simulink model "proc_control"  (R2024b)
settings: Solver=FixedStepAuto  StartTime=0.0  StopTime=inf  RelTol=1e-3
InitFcn:
  | InitProcControl;
model workspace (MAT data in the model file):
  SL_ROS_VariableLengthArrays_MaxSizes : object (value not decoded)
values from neighbouring files (symbols this model uses):
  A = T200Spec16V{:,3}    [InitProcControl.m]
  dmax = simulation.drift.nominal .* rand(1,6)    [InitProcControl.m]
  dmin = -simulation.drift.nominal .* rand(1,6)    [InitProcControl.m]
  dSeedX = round(rand*10)    [InitProcControl.m]
  dts = 5    [InitProcControl.m]
  N = T200Spec16V{:,6}    [InitProcControl.m]
  PWM = T200Spec16V{:,1}    [InitProcControl.m]
  RPM = T200Spec16V{:,2}    [InitProcControl.m]
undefined symbols (not defined in the file or in its folder): angular_velocity, current_gains, data, data_SL_Info, DiscIntNeverNeededParam, elevation, heading, is_mpc_alive, is_trajectory_done, linear_acceleration, motor1, motor2, motor3, motor4, motor5, motor6, motor7, motor8, MPC, mpc_mode, mpc_status, orientation, physics, pose, position, simulation, simulink, target_reached, thrusters_status, thrusters_status_SL_Info, twist, x_vel_btm, y_vel_btm, z_vel_btm
libraries: ros2lib x85, aerolibutil x12, simulink x9, mpclib x3, embmathops x2, sharedtransform x2, robotcorelib x2, sharedTrackingLibrary x1
(part 2 of 3)

== system proc_control/Subsystem Controller/If Action Subsystem ==
  mode : Inport
  mo : Inport  Port=2
  Current : Inport  Port=3
  mpcParams : Inport  Port=4
  Action Port : ActionPort  InitializeStates=reset  ActionPortLabel=if(u1 >= 0)
  Bus Creator : BusCreator  Inputs=9
  Bus Selector : BusSelector  OutputSignals=qS2W
  Bus Selector1 : BusSelector  OutputSignals=data
  Constant : Constant  Commented=on  Value=false
  MATLAB System : MATLABSystem  System=mpcManager  mpcConst=MPC  mode=mode  SimulateUsing=Code generation
      mask Type: mpcManager
      mask Display:
      | disp('mpcManager');
      | port_label('input',1,'newRosGains');
      | port_label('input',2,'rosGains');
      | port_label('input',3,'mode');
      | port_label('input',4,'newReadCurrent');
      | port_label('input',5,'readCurrent');
      | port_label('input',6,'estimatedCurrent');
      | port_label('input',7,'mo');
      | port_label('input',8,'mpcParams');
      | port_label('output',1,'mvmin');
      | port_label('output',2,'mvmax');
      | port_label('output',3,'ywt');
      | port_label('output',4,'mvwt');
      | port_label('output',5,'dmwwt');
      | port_label('output',6,'tInfo');
      | port_label('output',7,'kill');
      | port_label('output',8,'p');
      | port_label('output',9,'m');
  Subscribe : ros2lib/Subscribe  topicSource=Specify your own  topic=/proc_control/set_mpc_gains  messageType=sonia_common_ros2/MpcGains  sampleTime=inf  QOSHistory=Keep last  QOSDepth=1  QOSReliability=Reliable  QOSDurability=Volatile  QOSDeadline=5  QOSLifespan=5  QOSLiveliness=Automatic  QOSLeaseDuration=5  QOSAvoidROSNamespaceConventions=off
  Subscribe1 : ros2lib/Subscribe  topicSource=Specify your own  topic=/provider_power/current_not  messageType=std_msgs/Float64MultiArray  sampleTime=-1  QOSHistory=Keep last  QOSDepth=1  QOSReliability=Reliable  QOSDurability=Volatile  QOSDeadline=5  QOSLifespan=5  QOSLiveliness=Automatic  QOSLeaseDuration=5  QOSAvoidROSNamespaceConventions=off
  Subsystem : Subsystem  Commented=on
  Transpose : Math  Operator=transpose
  MPC param : Outport
  wires:
  mode/1 -> MATLAB System/3
  Current/1 -> MATLAB System/6
  mo/1 -> Bus Selector/1
  Transpose/1 -> MATLAB System/5
  Bus Selector1/1 -> Transpose/1  "<data>"
  Bus Selector/1 -> MATLAB System/7  "<qS2W>"
  MATLAB System/1 -> Bus Creator/1  "mvmin"
  MATLAB System/2 -> Bus Creator/2  "mvmax"
  MATLAB System/3 -> Bus Creator/3  "ywt"
  MATLAB System/4 -> Bus Creator/4  "mvwt"
  MATLAB System/5 -> Bus Creator/5  "dmwwt"
  MATLAB System/6 -> Bus Creator/6  "thrustersStatus"
  MATLAB System/7 -> Bus Creator/7  "kill"
  MATLAB System/8 -> Bus Creator/8  "p"
  MATLAB System/9 -> Bus Creator/9  "m"
  Bus Creator/1 -> MPC param/1
  mpcParams/1 -> MATLAB System/8
  Subscribe1/2 -> Bus Selector1/1  "data"
  Subscribe1/1 -> MATLAB System/4
  Subscribe/2 -> MATLAB System/2
  Subscribe/1 -> MATLAB System/1

== system proc_control/Subsystem Controller/Post Traitement ==
  In1 : Inport
  MpcParams : Inport  Port=2
  Bus Creator : BusCreator  Inputs=6
  Bus Selector : BusSelector  OutputSignals=mv
  Bus Selector1 : BusSelector  OutputSignals=mvmax,mvmin
  Bus Selector2 : BusSelector  OutputSignals=MpcStatus
  Bus Selector3 : BusSelector  OutputSignals=alive
  Data Type Conversion : DataTypeConversion  OutDataTypeStr=boolean  SaturateOnIntegerOverflow=off  RndMeth=Floor
  Delay : Delay  DelayLength=1  SampleTime=MPC.Ts
  N to A : Lookup_n-D  NumberOfTableDimensions=1  BreakpointsForDimension1=N  BreakpointsForDimension3=[5, 7]  BeginIndexSearchUsingPreviousIndexResult=on  Table=A  InterpMethod=Nearest  DiagnosticForOutOfRangeInput=Warning  RemoveProtectionInput=on  InternalRulePriority=Speed  OutDataTypeStr=uint16  RndMeth=Simplest
  PSU Safe : simulink/Discontinuities/Saturation Dynamic  OutMin=[]  OutMax=[]  OutDataTypeStr=Inherit: Same as second input  OutDataType=fixdt(1, 16)  OutScaling=2^-10  DoSatur=off
  Sum : Sum  Inputs=|+-
  Transpose : Math  Operator=transpose
  n-D Lookup Table1 : Lookup_n-D  NumberOfTableDimensions=1  BreakpointsForDimension1=N  BreakpointsForDimension3=[5, 7]  BeginIndexSearchUsingPreviousIndexResult=on  Table=PWM  InterpMethod=Nearest  DiagnosticForOutOfRangeInput=Warning  RemoveProtectionInput=on  InternalRulePriority=Speed  OutDataTypeStr=uint16  RndMeth=Simplest
  out : Outport
  wires:
  In1/1 -> Bus Selector3/1, Bus Selector2/1, Bus Selector/1
  Bus Selector/1 -> Transpose/1  "<mv>"
  Transpose/1 -> PSU Safe/2
  Bus Selector1/1 -> PSU Safe/1  "<mvmax>"
  Bus Selector1/2 -> PSU Safe/3  "<mvmin>"
  PSU Safe/1 -> N to A/1, n-D Lookup Table1/1, Bus Creator/3  "Newton"
  n-D Lookup Table1/1 -> Bus Creator/2  "pwm"
  N to A/1 -> Bus Creator/1  "current"
  MpcParams/1 -> Bus Creator/4, Bus Selector1/1  "mpcParams"
  Bus Selector2/1 -> Bus Creator/5  "<MpcStatus>"
  Bus Selector3/1 -> Sum/2, Delay/1  "<alive>"
  Delay/1 -> Sum/1
  Sum/1 -> Data Type Conversion/1
  Data Type Conversion/1 -> Bus Creator/6  "isMpcAlive"
  Bus Creator/1 -> out/1

== system proc_control/Subsystem ProcNav/AHRS//Detph Mesurments ==
  note: Modified with Zac
  note: REVIEW
  note: mettre le quaternion dans
      | le W frame
  y : Inport
  Bus Selector : BusSelector  OutputSignals=VN IMU Quaternion  OutputAsBus=on
  Bus Selector1 : BusSelector  OutputSignals=VN IMU Linear Acc  OutputAsBus=on
  Bus Selector2 : BusSelector  OutputSignals=VN IMU Angular Rate  OutputAsBus=on
  Constant : Constant  Value=simulation.sensors.imu.acc.bias
  Discrete-Time Integrator : DiscreteIntegrator  IntegratorMethod=Integration: Trapezoidal  SampleTime=-1  ICPrevOutput=DiscIntNeverNeededParam  ICPrevScaledInput=DiscIntNeverNeededParam
  MATLAB Function : MATLAB Function  TreatAsAtomicUnit=on
  Mux : Mux  Inputs=2
  Quaternion Conjugate : aerolibutil/Quaternion Conjugate
  Quaternion Inverse : aerolibutil/Quaternion Inverse
  Quaternion Rotation : aerolibutil/Quaternion Rotation
  Quaternion Rotation1 : aerolibutil/Quaternion Rotation
  Sum : Sum  Inputs=-+|
  IMU : Outport
  wires:
  y/1 -> Bus Selector2/1, Bus Selector1/1, Bus Selector/1
  Bus Selector/1 -> MATLAB Function/1(u), Quaternion Rotation1/1
  MATLAB Function/1(y) -> Quaternion Conjugate/1
  Quaternion Conjugate/1 -> Quaternion Rotation/1, Quaternion Inverse/1
  Quaternion Inverse/1 -> Mux/1  "qS2W"
  Quaternion Rotation1/1 -> Sum/1
  Bus Selector1/1 -> Quaternion Rotation/2, Sum/2
  Constant/1 -> Quaternion Rotation1/2
  Bus Selector2/1 -> Mux/2  "Angular Rate"
  Sum/1 -> Discrete-Time Integrator/1
  Mux/1 -> IMU/1

== system proc_control/Subsystem ProcNav/DVL Measurements ==
  note: Mettre les vitesse dvl dans le frame Sous-marin
  DVL Velocity : Inport
  mecConst : Inport  Port=2
  Enable : EnablePort
  Bus Creator : BusCreator  Inputs=3
  Bus Selector : BusSelector  OutputSignals=dvl_rotation
  Bus Selector1 : BusSelector  OutputSignals=DVL Bot Velocity
  Bus Selector2 : BusSelector  OutputSignals=DVL Water Velocity
  Constant : Constant  Value=simulation.sensors.dvl.maxSpeedThres
  DVL2Ship : Subsystem
  MATLAB Function : MATLAB Function  TreatAsAtomicUnit=on
  Quaternion Rotation : aerolibutil/Quaternion Rotation
  Scope : Scope
  DVL Measurements : Outport
  wires:
  mecConst/1 -> Bus Selector/1
  DVL Velocity/1 -> Bus Selector1/1, Bus Selector2/1
  Bus Selector/1 -> DVL2Ship/1(dvl Rotation)  "<dvl_rotation>"
  Bus Selector1/1 -> MATLAB Function/1(vBot)  "<DVL Bot Velocity>"
  Bus Selector2/1 -> MATLAB Function/2(vWater)  "<DVL Water Velocity>"
  Constant/1 -> MATLAB Function/3(thres)
  MATLAB Function/1(v) -> Quaternion Rotation/2
  DVL2Ship/1(Quat) -> Quaternion Rotation/1
  Quaternion Rotation/1 -> Bus Creator/1, Scope/1  "Body Velocity"
  MATLAB Function/2(error) -> Bus Creator/2  "error"
  MATLAB Function/3(enable) -> Bus Creator/3  "enable"
  Bus Creator/1 -> DVL Measurements/1

== system proc_control/Subsystem ProcNav/Depth Measurements ==
  note: Transformer la mesure du detph selon BF
  y : Inport
  mecConst : Inport  Port=2
  xhat : Inport  Port=3
  Enable : EnablePort
  Bus Selector : BusSelector  OutputSignals=Pressure Depth  OutputAsBus=on
  Bus Selector1 : BusSelector  OutputSignals=depth_pose
  Discrete Transfer Fcn : DiscreteTransferFcn  Numerator=[physics.thruster.a1 0 ]  Denominator="[1  physics.thruster.b0]"
  Discrete Derivative : simulink/Discrete/Discrete Derivative  gainval=1.0  ICPrevScaledInput=0.0  OutMin=[]  OutMax=[]  OutDataType=fixdt(1, 16)  OutScaling=2^-10  DoSatur=off
  Mux : Mux  Inputs=2
  Quaternion Rotation : aerolibutil/Quaternion Rotation
  Selector : Selector  InputPortWidth=7  IndexOptions=Index vector (dialog)  Indices=[1:4]  OutputSizes=1
  Selector1 : Selector  InputPortWidth=3  IndexOptions=Index vector (dialog)  Indices=[3]  OutputSizes=1
  Sum : Sum  Inputs=|+-
  Depth Measurements : Outport
  wires:
  y/1 -> Bus Selector/1
  Bus Selector/1 -> Sum/1  "pressure Depth"
  Sum/1 -> Mux/1, Discrete Derivative/1  "z position"
  xhat/1 -> Selector/1
  mecConst/1 -> Bus Selector1/1
  Selector/1 -> Quaternion Rotation/1
  Bus Selector1/1 -> Quaternion Rotation/2  "<depth_pose>"
  Quaternion Rotation/1 -> Selector1/1
  Selector1/1 -> Sum/2
  Mux/1 -> Depth Measurements/1
  Discrete Derivative/1 -> Discrete Transfer Fcn/1
  Discrete Transfer Fcn/1 -> Mux/2  "z velocity"

== system proc_control/Subsystem ProcNav/Enabled Subsystem ==
  stateFuncArguments : Inport
  AHRS Mesurments : Inport  Port=2
  "DVL Measurements " : Inport  Port=3
  Depth Measurements : Inport  Port=4
  mecConst : Inport  Port=5
  SLAM VIS : Inport  Port=6
  Enable : EnablePort  StatesWhenEnabling=reset
  Bus Selector : BusSelector  OutputSignals=dvl_lost_override
  Bus Selector1 : BusSelector  OutputSignals=enable,Body Velocity
  Bus Selector2 : BusSelector  OutputSignals=VisIsEnabled,VisData
  Constant : Constant
  Constant1 : Constant  Value=false
  Extended Kalman Filter : sharedTrackingLibrary/Extended Kalman Filter  StateTransitionFcn=EkfNavStatesEq  HasStateTransitionJacobianFcn=off  HasAdditiveProcessNoise=Additive  ProcessNoise=kalman.Cx  HasTimeVaryingProcessNoise=off  HasStateTransitionFcnExtraArgument=1  InitialState=kalman.Xi  InitialStateCovariance=kalman.Ci  MeasurementFcn1=EkfNavAhrs  HasMeasurementJacobianFcn1=off  HasMeasurementEnablePort1=off  HasAdditiveMeasurementNoise1=Additive  MeasurementNoise1=kalman.Cimu  HasTimeVaryingMeasurementNoise1=off  HasMeasurementFcnExtraArgument1=0  HasMeasurementWrapping1=off  MeasurementFcn2=EkfNavDvl  HasMeasurementJacobianFcn2=off  HasMeasurementEnablePort2=on  HasAdditiveMeasurementNoise2=Additive  MeasurementNoise2=kalman.Cdvl  HasTimeVaryingMeasurementNoise2=off  HasMeasurementFcnExtraArgument2=0  HasMeasurementWrapping2=off  MeasurementFcn3=EkfNavDepth  HasMeasurementJacobianFcn3=off  HasMeasurementEnablePort3=off  HasAdditiveMeasurementNoise3=Additive  MeasurementNoise3=kalman.Cdepth  HasTimeVaryingMeasurementNoise3=off  HasMeasurementFcnExtraArgument3=0  HasMeasurementWrapping3=off  MeasurementFcn4=EkfNavSlamVis  HasMeasurementJacobianFcn4=off  HasMeasurementEnablePort4=on  HasAdditiveMeasurementNoise4=Additive  MeasurementNoise4=kalman.CslamVis  HasTimeVaryingMeasurementNoise4=off  HasMeasurementFcnExtraArgument4=0  HasMeasurementWrapping4=off  MeasurementFcn5=EkfNavSlamTracking  HasMeasurementJacobianFcn5=off  HasMeasurementEnablePort5=on  HasAdditiveMeasurementNoise5=Additive  MeasurementNoise5=kalman.CslamTracking  HasTimeVaryingMeasurementNoise5=off  HasMeasurementFcnExtraArgument5=0  HasMeasurementWrapping5=off  EnableMultirate=on  StateTransitionFcnSampleTime=simulink.procNav.sampletime  MeasurementFcn1SampleTime=simulink.procNav.imuDepth.sampletime  MeasurementFcn2SampleTime=simulink.procNav.dvl.sampletime  MeasurementFcn3SampleTime=simulation.sensors.depth.sampletime  MeasurementFcn4SampleTime=0.1  MeasurementFcn5SampleTime=0.1  UseCurrentEstimator=on  OutputStateCovariance=off  DataType=double  SampleTime=1  NumberOfMeasurements=4
  Switch : Switch  Criteria=u2 > Threshold  SaturateOnIntegerOverflow=off  InputSameDT=off
  Zero-Order Hold : ZeroOrderHold  SampleTime=simulink.procNav.dvl.sampletime
  Zero-Order Hold1 : ZeroOrderHold  SampleTime=simulation.sensors.depth.sampletime
  xhat : Outport
  wires:
  stateFuncArguments/1 -> Extended Kalman Filter/1
  AHRS Mesurments/1 -> Extended Kalman Filter/2
  mecConst/1 -> Bus Selector/1
  Constant/1 -> Switch/1
  Bus Selector/1 -> Switch/2  "<dvl_lost_override>"
  "DVL Measurements "/1 -> Bus Selector1/1
  Bus Selector1/1 -> Switch/3  "<enable>"
  Bus Selector1/2 -> Zero-Order Hold/1  "<Body Velocity>"
  Zero-Order Hold/1 -> Extended Kalman Filter/4
  Depth Measurements/1 -> Zero-Order Hold1/1
  Zero-Order Hold1/1 -> Extended Kalman Filter/5
  Extended Kalman Filter/1 -> xhat/1
  SLAM VIS/1 -> Bus Selector2/1
  Bus Selector2/1 -> Extended Kalman Filter/6  "<VisIsEnabled>"
  Bus Selector2/2 -> Extended Kalman Filter/7  "<VisData>"
  Constant1/1 -> Extended Kalman Filter/3

== system proc_control/Subsystem ProcNav/Reset Logic ==
  In1 : Inport
  2 : Inport  Port=2
  AND : Logic  IconShape=distinctive  AllPortsSameDT=off  OutDataTypeStr=boolean
  NOT : Logic  Operator=NOT  IconShape=distinctive  AllPortsSameDT=off  OutDataTypeStr=boolean
  Out1 : Outport
  wires:
  2/1 -> AND/2
  In1/1 -> NOT/1
  NOT/1 -> AND/1
  AND/1 -> Out1/1

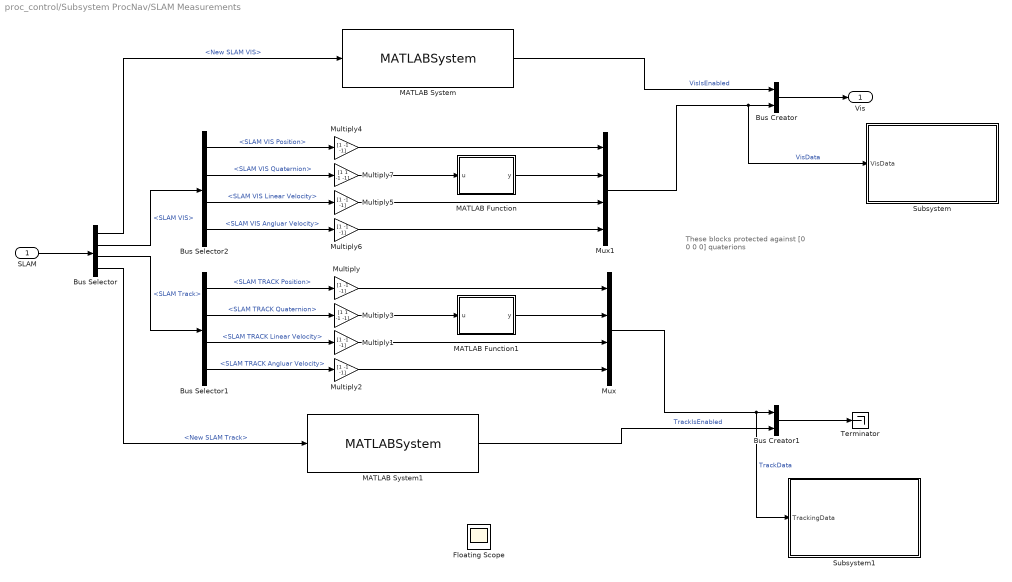
== system proc_control/Subsystem ProcNav/SLAM Measurements ==
  note: These blocks protected against
      | [0 0 0 0] quaterions
  SLAM : Inport
  Bus Creator : BusCreator  Inputs=2
  Bus Creator1 : BusCreator  Inputs=2
  Bus Selector : BusSelector  OutputSignals=New SLAM VIS,SLAM VIS,SLAM Track,New SLAM Track
  Bus Selector1 : BusSelector  OutputSignals=SLAM TRACK Position,SLAM TRACK Quaternion,SLAM TRACK Linear Velocity,SLAM TRACK Angluar Velocity
  Bus Selector2 : BusSelector  OutputSignals=SLAM VIS Position,SLAM VIS Quaternion,SLAM VIS Linear Velocity,SLAM VIS Angluar Velocity
  Floating Scope : Scope
      settings: Floating=on
  MATLAB Function : MATLAB Function  TreatAsAtomicUnit=on
  MATLAB Function1 : MATLAB Function  TreatAsAtomicUnit=on
  MATLAB System : MATLABSystem  System=SlamFreshCheck  timeoutCounter=7  SimulateUsing=Code generation
      mask Type: SlamFreshCheck
      mask Display:
      | disp('SlamFreshCheck');
      | port_label('input',1,'isNew');
      | port_label('output',1,'isEnabled');
  MATLAB System1 : MATLABSystem  System=SlamFreshCheck  timeoutCounter=3  SimulateUsing=Code generation
      mask Type: SlamFreshCheck
      mask Display:
      | disp('SlamFreshCheck');
      | port_label('input',1,'isNew');
      | port_label('output',1,'isEnabled');
  Multiply{,1..2,4..6} (6 alike) : Gain  Gain=[1 -1 -1]
  Multiply3 : Gain  Gain=[1 1 -1 -1]
  Multiply7 : Gain  Gain=[1 1 -1 -1]
  Mux : Mux
  Mux1 : Mux
  Subsystem : Subsystem
  Subsystem1 : Subsystem
  Terminator : Terminator
  Vis : Outport
  wires:
  SLAM/1 -> Bus Selector/1
  Bus Selector/2 -> Bus Selector2/1  "<SLAM VIS>"
  Bus Selector/3 -> Bus Selector1/1  "<SLAM Track>"
  Multiply2/1 -> Mux/4
  Multiply1/1 -> Mux/3
  Bus Selector1/2 -> Multiply3/1  "<SLAM TRACK Quaternion>"
  Bus Selector1/1 -> Multiply/1  "<SLAM TRACK Position>"
  Multiply/1 -> Mux/1
  Bus Selector1/3 -> Multiply1/1  "<SLAM TRACK Linear Velocity>"
  Multiply3/1 -> MATLAB Function1/1(u)
  Bus Selector1/4 -> Multiply2/1  "<SLAM TRACK Angluar Velocity>"
  Bus Selector2/3 -> Multiply5/1  "<SLAM VIS Linear Velocity>"
  Bus Selector2/4 -> Multiply6/1  "<SLAM VIS Angluar Velocity>"
  Bus Selector2/2 -> Multiply7/1  "<SLAM VIS Quaternion>"
  Mux1/1 -> Subsystem/1(VisData), Bus Creator/2  "VisData"
  Bus Selector2/1 -> Multiply4/1  "<SLAM VIS Position>"
  Mux/1 -> Subsystem1/1(TrackingData), Bus Creator1/1  "TrackData"
  Multiply4/1 -> Mux1/1
  Multiply6/1 -> Mux1/4
  Multiply7/1 -> MATLAB Function/1(u)
  Multiply5/1 -> Mux1/3
  MATLAB Function/1(y) -> Mux1/2
  MATLAB Function1/1(y) -> Mux/2
  Bus Selector/4 -> MATLAB System1/1  "<New SLAM Track>"
  Bus Selector/1 -> MATLAB System/1  "<New SLAM VIS>"
  MATLAB System/1 -> Bus Creator/1  "VisIsEnabled"
  Bus Creator/1 -> Vis/1
  Bus Creator1/1 -> Terminator/1
  MATLAB System1/1 -> Bus Creator1/2  "TrackIsEnabled"

== system proc_control/Subsystem ProcNav/State function arguments ==
  thrust : Inport
  mecConst : Inport  Port=2
  Bus Selector : BusSelector  OutputSignals=mass,volume,sub_height,I,rg,rb,cdl,cdq,added_mass,rho,g  OutputAsBus=on
  Bus Selector1 : BusSelector  OutputSignals=thrusters  OutputAsBus=on
  Bus to Vector : BusToVector
  Delay : Delay  DelayLength=1  InitialCondition=[0,0,0,0,0,0,0,0]
  Display : Display
  Mux : Mux
  Probe : Probe  ProbeSignalDimensions=on
  Reshape : Reshape
  Transpose : Math  Operator=transpose
  Zero-Order Hold : ZeroOrderHold  SampleTime=simulink.procNav.sampletime
  stateFuncArguments : Outport
  wires:
  mecConst/1 -> Bus Selector/1, Bus Selector1/1
  Bus Selector1/1 -> Transpose/1
  thrust/1 -> Probe/1, Delay/1
  Delay/1 -> Zero-Order Hold/1
  Bus Selector/1 -> Bus to Vector/1
  Bus to Vector/1 -> Mux/3
  Transpose/1 -> Reshape/1
  Probe/1 -> Mux/1
  Zero-Order Hold/1 -> Mux/2
  Reshape/1 -> Mux/4, Display/1
  Mux/1 -> stateFuncArguments/1

== system proc_control/Subsystem ProcNav/mux2Bus ==
  xhat : Inport
  Bus Creator : BusCreator  Inputs=5
  Quaternion Inverse : aerolibutil/Quaternion Inverse
  Scope{,1..3} (4 alike) : Scope
  Selector : Selector  InputPortWidth=13  IndexOptions=Index vector (dialog)  Indices=[1:3]  OutputSizes=1
  Selector1 : Selector  InputPortWidth=13  IndexOptions=Index vector (dialog)  Indices=[4:7]  OutputSizes=1
  Selector2 : Selector  InputPortWidth=13  IndexOptions=Index vector (dialog)  Indices=[8:10]  OutputSizes=1
  Selector3 : Selector  InputPortWidth=13  IndexOptions=Index vector (dialog)  Indices=[11:13]  OutputSizes=1
  states : Outport
  wires:
  xhat/1 -> Selector3/1, Selector2/1, Selector1/1, Selector/1
  Selector/1 -> Scope/1, Bus Creator/1  "WorldPosition"
  Selector3/1 -> Scope3/1, Bus Creator/5  "Angular Rate"
  Selector1/1 -> Scope1/1, Bus Creator/2, Quaternion Inverse/1  "qS2W"
  Selector2/1 -> Scope2/1, Bus Creator/4  "Body Velocity"
  Quaternion Inverse/1 -> Bus Creator/3  "qW2S"
  Bus Creator/1 -> states/1

== system proc_control/Subsystem Trajectory/IDLE ==
  Action Port : ActionPort  ActionPortLabel=default:
  Bus Creator : BusCreator  Inputs=4
  Constant : Constant  Value=[0,0,0.3,1,0,0,0,0,0,0,0,0,0]
  Constant1 : Constant  Value=MPC.p
  Constant2 : Constant  Value=false
  Constant3 : Constant  Value=false
  MATLAB Function : MATLAB Function  TreatAsAtomicUnit=on
  Selector : Selector  InputPortWidth=13  IndexOptions=Index vector (dialog)  Indices=[1:7]  OutputSizes=1
  Transpose : Math  Operator=transpose
  y : Outport
  wires:
  Constant/1 -> Transpose/1
  Transpose/1 -> Selector/1, MATLAB Function/1(matrix)
  Constant1/1 -> MATLAB Function/2(p)
  MATLAB Function/1(y) -> Bus Creator/1  "Reference"
  Selector/1 -> Bus Creator/4  "target"
  Constant2/1 -> Bus Creator/2  "isReached"
  Constant3/1 -> Bus Creator/3  "isTrajDone"
  Bus Creator/1 -> y/1

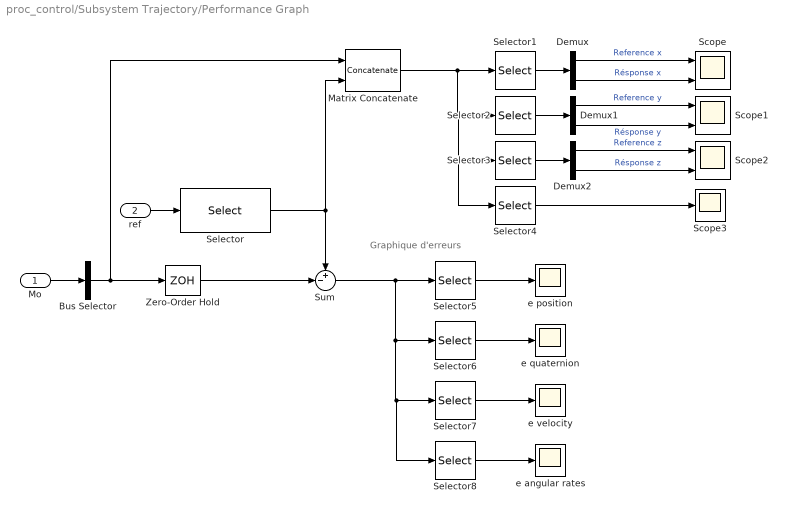
== system proc_control/Subsystem Trajectory/Performance Graph ==
  note: Graphique d'erreurs
  Mo : Inport
  ref : Inport  Port=2
  Bus Selector : BusSelector  OutputSignals=WorldPosition,qS2W,Body Velocity,Angular Rate  OutputAsBus=on
  Demux : Demux  Outputs=2
  Demux1 : Demux  Outputs=2
  Demux2 : Demux  Outputs=2
  Matrix Concatenate : Concatenate  Mode=Multidimensional array
  Scope : Scope  NumInputPorts=2
  Scope1 : Scope  NumInputPorts=2
  Scope2 : Scope  NumInputPorts=2
  Scope3 : Scope
  Selector : Selector  NumberOfDimensions=2  InputPortWidth=3  IndexOptions=Index vector (dialog),Index vector (dialog)  Indices=[1],[1:13]  OutputSizes=1,1
  Selector1 : Selector  NumberOfDimensions=2  InputPortWidth=3  IndexOptions=Index vector (dialog),Index vector (dialog)  Indices=[1:2],1  OutputSizes=1,1
  Selector2 : Selector  NumberOfDimensions=2  InputPortWidth=3  IndexOptions=Index vector (dialog),Index vector (dialog)  Indices=[1:2],2  OutputSizes=1,1
  Selector3 : Selector  NumberOfDimensions=2  InputPortWidth=3  IndexOptions=Index vector (dialog),Index vector (dialog)  Indices=[1:2],3  OutputSizes=1,1
  Selector4 : Selector  NumberOfDimensions=2  InputPortWidth=3  IndexOptions=Index vector (dialog),Index vector (dialog)  Indices=[1:2],[4:7]  OutputSizes=1,1
  Selector5 : Selector  InputPortWidth=13  IndexOptions=Index vector (dialog)  Indices=[1:3]  OutputSizes=1
  Selector6 : Selector  InputPortWidth=13  IndexOptions=Index vector (dialog)  Indices=[4:7]  OutputSizes=1
  Selector7 : Selector  InputPortWidth=13  IndexOptions=Index vector (dialog)  Indices=[8:10]  OutputSizes=1
  Selector8 : Selector  InputPortWidth=13  IndexOptions=Index vector (dialog)  Indices=[10:13]  OutputSizes=1
  Sum : Sum  Inputs=+-|
  Zero-Order Hold : ZeroOrderHold  SampleTime=-1
  e angular rates : Scope
  e position : Scope
  e quaternion : Scope
  e velocity : Scope
  wires:
  Mo/1 -> Bus Selector/1
  Bus Selector/1 -> Matrix Concatenate/1, Zero-Order Hold/1
  Zero-Order Hold/1 -> Sum/2
  ref/1 -> Selector/1
  Selector/1 -> Sum/1, Matrix Concatenate/2
  Matrix Concatenate/1 -> Selector4/1, Selector3/1, Selector2/1, Selector1/1
  Selector1/1 -> Demux/1
  Selector2/1 -> Demux1/1
  Selector3/1 -> Demux2/1
  Demux/1 -> Scope/1  "Reference x"
  Demux/2 -> Scope/2  "Résponse x"
  Demux1/1 -> Scope1/1  "Reference y"
  Demux1/2 -> Scope1/2  "Résponse y"
  Demux2/1 -> Scope2/1  "Reference z"
  Demux2/2 -> Scope2/2  "Résponse z"
  Selector4/1 -> Scope3/1
  Sum/1 -> Selector8/1, Selector7/1, Selector6/1, Selector5/1
  Selector5/1 -> e position/1
  Selector6/1 -> e quaternion/1
  Selector7/1 -> e velocity/1
  Selector8/1 -> e angular rates/1

== system proc_control/Subsystem Trajectory/ProcPlanner Trajectory ==
  isNew : Inport
  trajMsg : Inport  Port=2
  output : Inport  Port=3
  reset : Inport  Port=4
  rosParam : Inport  Port=5
  Action Port : ActionPort  ActionPortLabel=case [ 10 ]:
  Bus Creator : BusCreator  Inputs=4
  Bus Selector : BusSelector  OutputSignals=WorldPosition,qS2W,Body Velocity,Angular Rate  OutputAsBus=on
  Detect Rise Positive : simulink/Logic and Bit Operations/Detect Rise Positive  vinit=0  OutDataTypeStr=boolean
  MATLAB System : MATLABSystem  System=ProcPlannerManager  mpcConst=MPC  SimulateUsing=Code generation
      mask Type: ProcPlannerManager
      mask Display:
      | disp('ProcPlannerManager');
      | port_label('input',1,'isNew');
      | port_label('input',2,'trajMsg');
      | port_label('input',3,'reset');
      | port_label('input',4,'mesuredPose');
      | port_label('input',5,'mpcParams');
      | port_label('output',1,'currentPose');
      | port_label('output',2,'isReached');
      | port_label('output',3,'isTrajDone');
      | port_label('output',4,'initWpt');
  Refrence : Outport
  wires:
  isNew/1 -> Detect Rise Positive/1
  Detect Rise Positive/1 -> MATLAB System/1
  trajMsg/1 -> MATLAB System/2
  reset/1 -> MATLAB System/3
  output/1 -> Bus Selector/1
  Bus Selector/1 -> MATLAB System/4
  rosParam/1 -> MATLAB System/5
  MATLAB System/4 -> Bus Creator/4  "target"
  MATLAB System/3 -> Bus Creator/3  "isTrajDone"
  MATLAB System/2 -> Bus Creator/2  "isReached"
  MATLAB System/1 -> Bus Creator/1  "Reference"
  Bus Creator/1 -> Refrence/1

== system proc_control/Subsystem Trajectory/Send Current Target ==
  pose : Inport
  Blank Message : ros2lib/Blank Message  messageClass=Message  entityType=geometry_msgs/Pose  messageType=geometry_msgs/Pose  SampleTime=inf
  Bus Assignment : BusAssignment  AssignedSignals=position.x,position.y,position.z,orientation.w,orientation.x,orientation.y,orientation.z
  Demux : Demux  Outputs=7
  Publish : ros2lib/Publish  topicSource=Specify your own  topic=/proc_control/current_target  messageType=geometry_msgs/Pose  QOSHistory=Keep last  QOSDepth=1  QOSReliability=Reliable  QOSDurability=Volatile  QOSDeadline=Inf  QOSLifespan=5  QOSLiveliness=Automatic  QOSLeaseDuration=5  QOSAvoidROSNamespaceConventions=off
  Zero-Order Hold : ZeroOrderHold
  wires:
  Blank Message/1 -> Bus Assignment/1
  pose/1 -> Demux/1
  Demux/1 -> Bus Assignment/2
  Demux/2 -> Bus Assignment/3
  Demux/3 -> Bus Assignment/4
  Demux/4 -> Bus Assignment/5
  Demux/5 -> Bus Assignment/6
  Demux/6 -> Bus Assignment/7
  Demux/7 -> Bus Assignment/8
  Bus Assignment/1 -> Zero-Order Hold/1
  Zero-Order Hold/1 -> Publish/1

== system proc_control/Subsystem Trajectory/SpaceNav ==
  y : Inport
  Action Port : ActionPort  ActionPortLabel=case [ 19 20 21 ]:
  Bus Creator : BusCreator  Inputs=4
  Constant : Constant  Value=[0 0 0 1 0 0 0]
  Constant1 : Constant  Value=MPC.p
  Constant2 : Constant  Value=false  VectorParams1D=off
  Constant3 : Constant  Value=false  VectorParams1D=off
  MATLAB Function : MATLAB Function  TreatAsAtomicUnit=on
  Mux : Mux  Inputs=2
  Selector : Selector  InputPortWidth=13  IndexOptions=Index vector (dialog)  Indices=[1:7]  OutputSizes=1
  Transpose : Math  Operator=transpose  OutputSignalType=real
  Out1 : Outport
  wires:
  Constant/1 -> Mux/1
  y/1 -> Mux/2
  Mux/1 -> Transpose/1
  Transpose/1 -> Selector/1, MATLAB Function/1(matrix)
  Constant1/1 -> MATLAB Function/2(p)
  MATLAB Function/1(y) -> Bus Creator/1  "Reference"
  Selector/1 -> Bus Creator/4  "target"
  Constant3/1 -> Bus Creator/3  "isTrajDone"
  Constant2/1 -> Bus Creator/2  "isReached"
  Bus Creator/1 -> Out1/1

== system proc_control/Subsystem Trajectory/Subsystem ==
  Bus Selector : BusSelector  OutputSignals=linear.x,linear.y,linear.z  OutputAsBus=on
  Bus Selector1 : BusSelector  OutputSignals=angular.x,angular.y,angular.z  OutputAsBus=on
  Bus to Vector : BusToVector
  Bus to Vector1 : BusToVector
  Gain : Gain  Gain=-1
  Mux : Mux  Inputs=2
  Scope : Scope
  Subscribe : ros2lib/Subscribe  topicSource=Specify your own  topic=/spacenav/twist  messageType=geometry_msgs/Twist  sampleTime=1/25  QOSHistory=Keep last  QOSDepth=1  QOSReliability=Reliable  QOSDurability=Volatile  QOSDeadline=Inf  QOSLifespan=5  QOSLiveliness=Automatic  QOSLeaseDuration=5  QOSAvoidROSNamespaceConventions=off
  Terminator : Terminator
  y : Outport
  wires:
  Subscribe/1 -> Terminator/1
  Subscribe/2 -> Bus Selector1/1, Bus Selector/1
  Bus Selector/1 -> Bus to Vector/1
  Bus Selector1/1 -> Bus to Vector1/1
  Bus to Vector1/1 -> Gain/1
  Bus to Vector/1 -> Mux/1
  Gain/1 -> Mux/2
  Mux/1 -> Scope/1, y/1

== system proc_control/Subsystem Trajectory/Subsystem1 ==
  Subscribe : ros2lib/Subscribe  topicSource=Specify your own  topic=/proc_planner/send_trajectory_list  messageType=trajectory_msgs/MultiDOFJointTrajectoryPoint  sampleTime=2  QOSHistory=Keep last  QOSDepth=1  QOSReliability=Reliable  QOSDurability=Volatile  QOSDeadline=Inf  QOSLifespan=5  QOSLiveliness=Automatic  QOSLeaseDuration=5  QOSAvoidROSNamespaceConventions=off
  isNew : Outport
  trajMsg : Outport  Port=2
  wires:
  Subscribe/1 -> isNew/1
  Subscribe/2 -> trajMsg/1

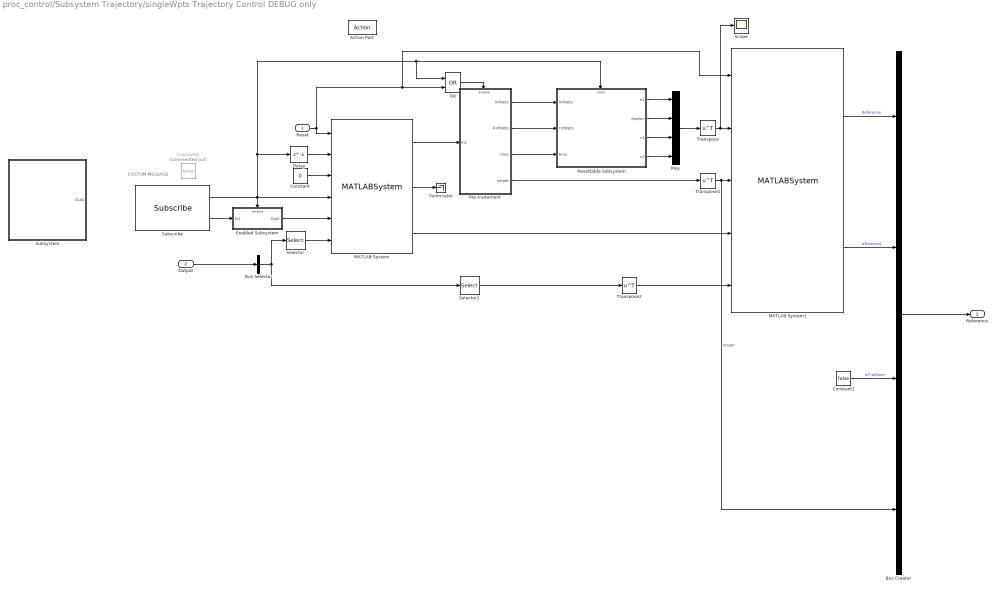
== system proc_control/Subsystem Trajectory/singleWpts Trajectory Control DEBUG only ==
  note: CUSTOM MESSAGE
  Reset : Inport
  Output : Inport  Port=2
  Action Port : ActionPort  InitializeStates=reset  ActionPortLabel=case [ 11 30 31 40 41 ]:
  Bus Creator : BusCreator  Inputs=4
  Bus Selector : BusSelector  OutputSignals=WorldPosition,qS2W,Body Velocity,Angular Rate  OutputAsBus=on
  Constant : Constant  Value=0
  Constant1 : Constant  Value=false
  Constant2 : Constant  Commented=on  Value=false
  Delay : Delay  DelayLength=1
  Enabled Subsystem : Subsystem  TreatAsAtomicUnit=on
  MATLAB System : MATLABSystem  System=AddPose  buffSize=2  elementSize=9  SimulateUsing=Code generation
      mask Type: AddPose
      mask Display:
      | disp('AddPose');
      | port_label('input',1,'reset');
      | port_label('input',2,'compute');
      | port_label('input',3,'clearBuffer');
      | port_label('input',4,'isNew');
      | port_label('input',5,'waypoint');
      | port_label('input',6,'xk');
      | port_label('output',1,'waypoints');
      | port_label('output',2,'count');
      | port_label('output',3,'initCond');
  MATLAB System1 : MATLABSystem  System=TrajectoryManager  SampleTime=MPC.Ts  OffsetTime=0  prediction=MPC.p  bufferSize=6001  linearConvergence=.25  quaternionConvergence=.22  TargetThreshold=2  SimulateUsing=Code generation
      mask Type: TrajectoryManager
      mask Display:
      | disp('TrajectoryManager');
      | port_label('input',1,'reset');
      | port_label('input',2,'poses');
      | port_label('input',3,'target');
      | port_label('input',4,'x0');
      | port_label('input',5,'mesuredPose');
      | port_label('output',1,'currentPose');
      | port_label('output',2,'isReached');
  Mux : Mux
  OR : Logic  Operator=OR  IconShape=distinctive  AllPortsSameDT=off  OutDataTypeStr=boolean
  Pre-traitement : Subsystem  TreatAsAtomicUnit=on
  Resettable Subsystem : Subsystem  TreatAsAtomicUnit=on
  Scope : Scope
  Selector : Selector  InputPortWidth=13  IndexOptions=Index vector (dialog)  Indices=[1:7]  OutputSizes=1
  Selector1 : Selector  InputPortWidth=13  IndexOptions=Index vector (dialog)  Indices=[1:13]  OutputSizes=1
  Subscribe : ros2lib/Subscribe  topicSource=Specify your own  topic=/proc_control/add_pose  messageType=sonia_common_ros2/Pose  sampleTime=-1  QOSHistory=Keep last  QOSDepth=1  QOSReliability=Reliable  QOSDurability=Volatile  QOSDeadline=Inf  QOSLifespan=5  QOSLiveliness=Automatic  QOSLeaseDuration=inf  QOSAvoidROSNamespaceConventions=off
  Subsystem : Subsystem
  Terminator : Terminator
  Transpose : Math  Operator=transpose
  Transpose1 : Math  Operator=transpose
  Transpose2 : Math  Operator=transpose
  Reference : Outport
  wires:
  Reset/1 -> MATLAB System1/1, OR/2, MATLAB System/1
  Subscribe/1 -> Resettable Subsystem/Reset, OR/1, Delay/1, Enabled Subsystem/Enable, MATLAB System/4
  Enabled Subsystem/1(Out1) -> MATLAB System/5
  Constant/1 -> MATLAB System/3
  Delay/1 -> MATLAB System/2
  MATLAB System/2 -> Terminator/1
  Output/1 -> Bus Selector/1
  Bus Selector/1 -> Selector/1, Selector1/1
  Selector/1 -> MATLAB System/6
  MATLAB System/1 -> Pre-traitement/1(In1)
  OR/1 -> Pre-traitement/Enable
  Pre-traitement/1(linWpts) -> Resettable Subsystem/1(linWpts)
  Pre-traitement/2(RotWpts) -> Resettable Subsystem/2(rotWpts)
  Pre-traitement/3(time) -> Resettable Subsystem/3(time)
  Resettable Subsystem/1(n1) -> Mux/1
  Resettable Subsystem/2(epsilon) -> Mux/2
  Resettable Subsystem/3(v1) -> Mux/3
  Resettable Subsystem/4(v2) -> Mux/4
  Mux/1 -> Transpose/1
  Transpose/1 -> Scope/1, MATLAB System1/2
  Pre-traitement/4(target) -> Transpose1/1
  Transpose1/1 -> Bus Creator/4, MATLAB System1/3  "target"
  MATLAB System/3 -> MATLAB System1/4
  Transpose2/1 -> MATLAB System1/5
  Selector1/1 -> Transpose2/1
  MATLAB System1/1 -> Bus Creator/1  "Reference"
  MATLAB System1/2 -> Bus Creator/2  "isReached"
  Constant1/1 -> Bus Creator/3  "isTrajDone"
  Bus Creator/1 -> Reference/1
  Subscribe/2 -> Enabled Subsystem/1(In1)

== system proc_control/Enabled Subsystem/Send auv states/bus2mux ==
  Input : Inport
  Bus Selector : BusSelector  OutputSignals=WorldPosition,qS2W,Body Velocity,Angular Rate
  Mux : Mux
  states : Outport
  wires:
  Bus Selector/1 -> Mux/1  "<WorldPosition>"
  Input/1 -> Bus Selector/1
  Bus Selector/2 -> Mux/2  "<qS2W>"
  Mux/1 -> states/1
  Bus Selector/3 -> Mux/3  "<Body Velocity>"
  Bus Selector/4 -> Mux/4  "<Angular Rate>"

== system proc_control/Model System/Modele Thruster (Approximation)/Send RPM to unity ==
  In1 : Inport
  Blank Message : ros2lib/Blank Message  messageClass=Message  entityType=std_msgs/Int16MultiArray  messageType=std_msgs/Int16MultiArray  SampleTime=inf
  Bus Assignment : BusAssignment  AssignedSignals=data,data_SL_Info.CurrentLength
  Constant : Constant  Value=uint32(8)  VectorParams1D=off
  Constant1 : Constant  Value=int16(zeros(1,120))
  N to RPM : Lookup_n-D  NumberOfTableDimensions=1  BreakpointsForDimension1=N  BreakpointsForDimension3=[5, 7]  BreakpointsForDimension1DataTypeStr=double  BeginIndexSearchUsingPreviousIndexResult=on  Table=RPM  TableDataTypeStr=double  InterpMethod=Nearest  InternalRulePriority=Speed  OutDataTypeStr=int16  RndMeth=Simplest
  Product : Product  OutDataTypeStr=int16
  Publish : ros2lib/Publish  topicSource=Specify your own  topic=/proc_simulation/thruster_rpm  messageType=std_msgs/Int16MultiArray  QOSHistory=Keep last  QOSDepth=1  QOSReliability=Reliable  QOSDurability=Volatile  QOSDeadline=5  QOSLifespan=5  QOSLiveliness=Automatic  QOSLeaseDuration=5  QOSAvoidROSNamespaceConventions=off
  Sign : Signum
  Vector Concatenate : Concatenate
  wires:
  Blank Message/1 -> Bus Assignment/1
  Sign/1 -> Product/2
  In1/1 -> N to RPM/1, Sign/1
  N to RPM/1 -> Product/1
  Constant/1 -> Bus Assignment/3
  Bus Assignment/1 -> Publish/1
  Product/1 -> Vector Concatenate/1
  Constant1/1 -> Vector Concatenate/2
  Vector Concatenate/1 -> Bus Assignment/2

== system proc_control/Model System/Modele Thruster (Approximation)/T1 ==
  In1 : Inport
  Discrete Transfer Fcn : DiscreteTransferFcn  Numerator=[physics.thruster.a1 0 ]  Denominator="[1  physics.thruster.b0]"
  Out1 : Outport
  wires:
  In1/1 -> Discrete Transfer Fcn/1
  Discrete Transfer Fcn/1 -> Out1/1

== system proc_control/Model System/Modele Thruster (Approximation)/T2 ==
  In1 : Inport
  Discrete Transfer Fcn : DiscreteTransferFcn  Numerator=[physics.thruster.a1 0 ]  Denominator="[1  physics.thruster.b0]"
  Out1 : Outport
  wires:
  In1/1 -> Discrete Transfer Fcn/1
  Discrete Transfer Fcn/1 -> Out1/1

== system proc_control/Model System/Modele Thruster (Approximation)/T3 ==
  In1 : Inport
  Discrete Transfer Fcn : DiscreteTransferFcn  Numerator=[physics.thruster.a1 0 ]  Denominator="[1  physics.thruster.b0]"
  Out1 : Outport
  wires:
  In1/1 -> Discrete Transfer Fcn/1
  Discrete Transfer Fcn/1 -> Out1/1

== system proc_control/Model System/Modele Thruster (Approximation)/T4 ==
  In1 : Inport
  Discrete Transfer Fcn : DiscreteTransferFcn  Numerator=[physics.thruster.a1 0 ]  Denominator="[1  physics.thruster.b0]"
  Out1 : Outport
  wires:
  In1/1 -> Discrete Transfer Fcn/1
  Discrete Transfer Fcn/1 -> Out1/1

== system proc_control/Model System/Modele Thruster (Approximation)/T5 ==
  In1 : Inport
  Discrete Transfer Fcn : DiscreteTransferFcn  Numerator=[physics.thruster.a1 0 ]  Denominator="[1  physics.thruster.b0]"
  Out1 : Outport
  wires:
  In1/1 -> Discrete Transfer Fcn/1
  Discrete Transfer Fcn/1 -> Out1/1

== system proc_control/Model System/Modele Thruster (Approximation)/T6 ==
  In1 : Inport
  Discrete Transfer Fcn : DiscreteTransferFcn  Numerator=[physics.thruster.a1 0 ]  Denominator="[1  physics.thruster.b0]"
  Out1 : Outport
  wires:
  In1/1 -> Discrete Transfer Fcn/1
  Discrete Transfer Fcn/1 -> Out1/1

== system proc_control/Model System/Modele Thruster (Approximation)/T7 ==
  In1 : Inport
  Discrete Transfer Fcn : DiscreteTransferFcn  Numerator=[physics.thruster.a1 0 ]  Denominator="[1  physics.thruster.b0]"
  Out1 : Outport
  wires:
  In1/1 -> Discrete Transfer Fcn/1
  Discrete Transfer Fcn/1 -> Out1/1

== system proc_control/Model System/Modele Thruster (Approximation)/T8 ==
  In1 : Inport
  Discrete Transfer Fcn : DiscreteTransferFcn  Numerator=[physics.thruster.a1 0 ]  Denominator="[1  physics.thruster.b0]"
  Out1 : Outport
  wires:
  In1/1 -> Discrete Transfer Fcn/1
  Discrete Transfer Fcn/1 -> Out1/1

== system proc_control/Model System/Sensor Model/Hydrophones Model ==
  Output Variables : Inport
  Bus S elector : BusSelector  OutputSignals=x.World Position,x.Quaternion
  If : If  IfExpression=u1 == 0  ShowElse=off
  If Action Subsystem : Subsystem  TreatAsAtomicUnit=on
  MATLAB System : MATLABSystem  System=HydroModel  Physics=physics  simulation=simulation  pingerStartPosition=[10 0 5]  SimulateUsing=Code generation
      mask Type: HydroModel
      mask Display:
      | disp('HydroModel');
      | port_label('input',1,'isNewPosition');
      | port_label('input',2,'pingerPosition');
      | port_label('input',3,'worldPosition');
      | port_label('input',4,'quaternion');
      | port_label('output',1,'HydroMesurements');
  Publish : ros2lib/Publish  topicSource=Specify your own  topic=/proc_simulation/pinger_location  messageType=geometry_msgs/Vector3  QOSHistory=Keep last  QOSDepth=1  QOSReliability=Reliable  QOSDurability=Volatile  QOSDeadline=5  QOSLifespan=5  QOSLiveliness=Automatic  QOSLeaseDuration=5  QOSAvoidROSNamespaceConventions=off
  Subscribe : ros2lib/Subscribe  topicSource=Specify your own  topic=/proc_simulation/set_pinger_location  messageType=geometry_msgs/Vector3  sampleTime=-1  QOSHistory=Keep last  QOSDepth=1  QOSReliability=Reliable  QOSDurability=Volatile  QOSDeadline=5  QOSLifespan=5  QOSLiveliness=Automatic  QOSLeaseDuration=5  QOSAvoidROSNamespaceConventions=off
  Zero-Order Hold : ZeroOrderHold
  Out1 : Outport
  wires:
  MATLAB System/1 -> Out1/1
  Subscribe/1 -> MATLAB System/1, If/1
  Subscribe/2 -> MATLAB System/2, If Action Subsystem/1(In1)
  Output Variables/1 -> Bus S elector/1
  If/1 -> If Action Subsystem/Action
  Bus S elector/1 -> MATLAB System/3  "<World Position>"
  If Action Subsystem/1(Out1) -> Zero-Order Hold/1
  Bus S elector/2 -> MATLAB System/4  "<Quaternion>"
  Zero-Order Hold/1 -> Publish/1

== system proc_control/Ros Command/Get_ROS_param/MPC Parameters ==
  Bus Creator : BusCreator  Inputs=2  OutDataTypeStr=Bus: mpcParams
  MPC Gains : Subsystem
  targetReached Params : Subsystem
  mpcParams : Outport
  wires:
  MPC Gains/1(gains) -> Bus Creator/1
  targetReached Params/1(targetReached) -> Bus Creator/2
  Bus Creator/1 -> mpcParams/1  "mpcParams"

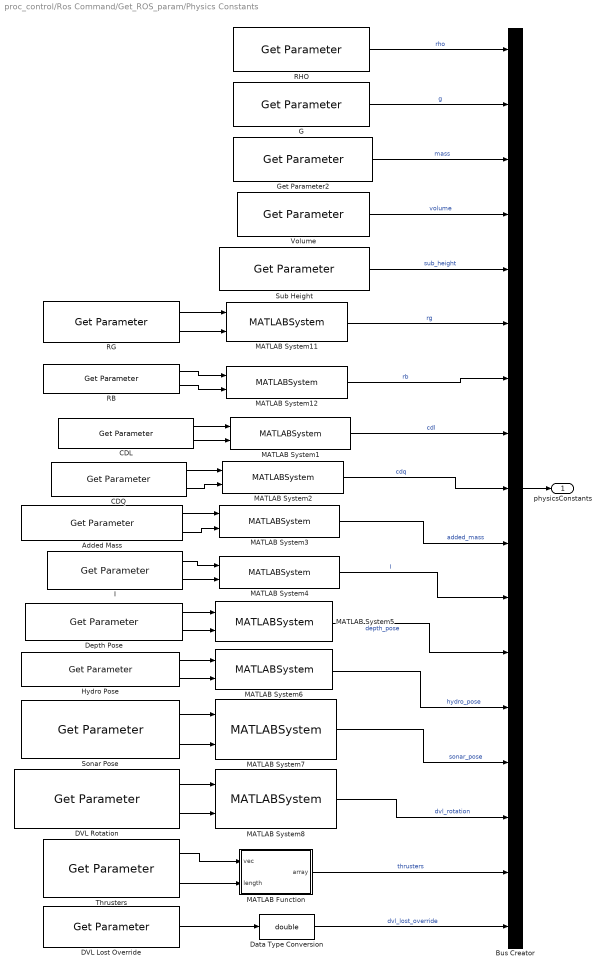
== system proc_control/Ros Command/Get_ROS_param/Physics Constants ==
  Added Mass : ros2lib/Get Parameter  ParameterName=proc_control.physics.added_mass  ParameterType=double[]  ParameterMaxArrayLength=64  ParameterInitialValue=int8([0,0,0,0,0,0])  SampleTime=-1  ModelName=proc_control  BlockId=ParamGet_proc_control_180
  Bus Creator : BusCreator  Inputs=17  OutDataTypeStr=Bus: physicsConstants  NonVirtualBus=on
  CDL : ros2lib/Get Parameter  ParameterName=proc_control.physics.cdl  ParameterType=double[]  ParameterMaxArrayLength=64  ParameterInitialValue=int8([0,0,0,0,0,0])  SampleTime=-1  ModelName=proc_control  BlockId=ParamGet_proc_control_175
  CDQ : ros2lib/Get Parameter  ParameterName=proc_control.physics.cdq  ParameterType=double[]  ParameterMaxArrayLength=64  ParameterInitialValue=int8([0,0,0,0,0,0])  SampleTime=-1  ModelName=proc_control  BlockId=ParamGet_proc_control_177
  DVL Lost Override : ros2lib/Get Parameter  ParameterName=proc_control.physics.dvl_lost_override  ParameterType=boolean  ParameterMaxArrayLength=16  ParameterInitialValue=true  SampleTime=-1  ModelName=proc_control  BlockId=ParamGet_proc_control_196
  DVL Rotation : ros2lib/Get Parameter  ParameterName=proc_control.physics.dvl_rotation  ParameterType=double[]  ParameterMaxArrayLength=64  ParameterInitialValue=int8([0,0,0])  SampleTime=-1  ModelName=proc_control  BlockId=ParamGet_proc_control_192
  Data Type Conversion : DataTypeConversion  OutDataTypeStr=double  SaturateOnIntegerOverflow=off  RndMeth=Floor
  Depth Pose : ros2lib/Get Parameter  ParameterName=proc_control.physics.depth_pose  ParameterType=double[]  ParameterMaxArrayLength=64  ParameterInitialValue=int8([0,0,0])  SampleTime=-1  ModelName=proc_control  BlockId=ParamGet_proc_control_184
  G : ros2lib/Get Parameter  ParameterName=proc_control.physics.g  ParameterType=double  ParameterMaxArrayLength=16  ParameterInitialValue=physics.g  SampleTime=-1  ModelName=proc_control  BlockId=ParamGet_proc_control_167
  Get Parameter2 : ros2lib/Get Parameter  ParameterName=proc_control.physics.mass  ParameterType=double  ParameterMaxArrayLength=16  ParameterInitialValue=physics.mass  SampleTime=-1  ModelName=proc_control  BlockId=ParamGet_proc_control_168
  Hydro Pose : ros2lib/Get Parameter  ParameterName=proc_control.physics.hydro_pose  ParameterType=double[]  ParameterMaxArrayLength=64  ParameterInitialValue=int8([0,0,0])  SampleTime=-1  ModelName=proc_control  BlockId=ParamGet_proc_control_186
  I : ros2lib/Get Parameter  ParameterName=proc_control.physics.I  ParameterType=double[]  ParameterMaxArrayLength=128  ParameterInitialValue=int8([0,0,0,0,0,0,0,0,0])  SampleTime=-1  ModelName=proc_control  BlockId=ParamGet_proc_control_182
  MATLAB Function : MATLAB Function  TreatAsAtomicUnit=on
  MATLAB System1 : MATLABSystem  System=Vector2DoubleArray  arraySize=[1, 6]  constantName='Linear drag constant'  SimulateUsing=Code generation
      mask Type: Vector2DoubleArray
      mask Display:
      | disp('Vector2DoubleArray');
      | port_label('input',1,'vector');
      | port_label('input',2,'length');
      | port_label('output',1,'array');
  MATLAB System11 : MATLABSystem  System=Vector2DoubleArray  arraySize=[1 3]  constantName='Center of Mass'  SimulateUsing=Code generation
      mask Type: Vector2DoubleArray
      mask Display:
      | disp('Vector2DoubleArray');
      | port_label('input',1,'vector');
      | port_label('input',2,'length');
      | port_label('output',1,'array');
  MATLAB System12 : MATLABSystem  System=Vector2DoubleArray  arraySize=[1, 3]  constantName='Center of Buoyancy'  SimulateUsing=Code generation
      mask Type: Vector2DoubleArray
      mask Display:
      | disp('Vector2DoubleArray');
      | port_label('input',1,'vector');
      | port_label('input',2,'length');
      | port_label('output',1,'array');
  MATLAB System2 : MATLABSystem  System=Vector2DoubleArray  arraySize=[1, 6]  constantName='Quadratic drag constant'  SimulateUsing=Code generation
      mask Type: Vector2DoubleArray
      mask Display:
      | disp('Vector2DoubleArray');
      | port_label('input',1,'vector');
      | port_label('input',2,'length');
      | port_label('output',1,'array');
  MATLAB System3 : MATLABSystem  System=Vector2DoubleArray  arraySize=[1, 6]  constantName='Added Mass'  SimulateUsing=Code generation
      mask Type: Vector2DoubleArray
      mask Display:
      | disp('Vector2DoubleArray');
      | port_label('input',1,'vector');
      | port_label('input',2,'length');
      | port_label('output',1,'array');
  MATLAB System4 : MATLABSystem  System=Vector2DoubleArray  arraySize=[1,9]  constantName='Inertia Tensor'  SimulateUsing=Code generation
      mask Type: Vector2DoubleArray
      mask Display:
      | disp('Vector2DoubleArray');
      | port_label('input',1,'vector');
      | port_label('input',2,'length');
      | port_label('output',1,'array');
  MATLAB System5 : MATLABSystem  System=Vector2DoubleArray  arraySize=[1 3]  constantName='Depth Pose'  SimulateUsing=Code generation
      mask Type: Vector2DoubleArray
      mask Display:
      | disp('Vector2DoubleArray');
      | port_label('input',1,'vector');
      | port_label('input',2,'length');
      | port_label('output',1,'array');
  MATLAB System6 : MATLABSystem  System=Vector2DoubleArray  arraySize=[1, 3]  constantName='Hydro Pose'  SimulateUsing=Code generation
      mask Type: Vector2DoubleArray
      mask Display:
      | disp('Vector2DoubleArray');
      | port_label('input',1,'vector');
      | port_label('input',2,'length');
      | port_label('output',1,'array');
  MATLAB System7 : MATLABSystem  System=Vector2DoubleArray  arraySize=[1, 3]  constantName='Sonar Pose'  SimulateUsing=Code generation
      mask Type: Vector2DoubleArray
      mask Display:
      | disp('Vector2DoubleArray');
      | port_label('input',1,'vector');
      | port_label('input',2,'length');
      | port_label('output',1,'array');
  MATLAB System8 : MATLABSystem  System=Vector2DoubleArray  arraySize=[1, 3]  constantName='DVL Rotation'  SimulateUsing=Code generation
      mask Type: Vector2DoubleArray
      mask Display:
      | disp('Vector2DoubleArray');
      | port_label('input',1,'vector');
      | port_label('input',2,'length');
      | port_label('output',1,'array');
  RB : ros2lib/Get Parameter  ParameterName=proc_control.physics.rb  ParameterType=double[]  ParameterMaxArrayLength=64  ParameterInitialValue=int8([0,0,0])  SampleTime=-1  ModelName=proc_control  BlockId=ParamGet_proc_control_173
  RG : ros2lib/Get Parameter  ParameterName=proc_control.physics.rg  ParameterType=double[]  ParameterMaxArrayLength=64  ParameterInitialValue=double([0,0,0])  SampleTime=-1  ModelName=proc_control  BlockId=ParamGet_proc_control_171
  RHO : ros2lib/Get Parameter  ParameterName=proc_control.physics.rho  ParameterType=double  ParameterMaxArrayLength=16  ParameterInitialValue=physics.rho  SampleTime=-1  ModelName=proc_control  BlockId=ParamGet_proc_control_166
  Sonar Pose : ros2lib/Get Parameter  ParameterName=proc_control.physics.sonar_pose  ParameterType=double[]  ParameterMaxArrayLength=64  ParameterInitialValue=int8([0,0,0])  SampleTime=-1  ModelName=proc_control  BlockId=ParamGet_proc_control_190
  Sub Height : ros2lib/Get Parameter  ParameterName=proc_control.physics.sub_height  ParameterType=double  ParameterMaxArrayLength=16  ParameterInitialValue=physics.height  SampleTime=-1  ModelName=proc_control  BlockId=ParamGet_proc_control_170
  Thrusters : ros2lib/Get Parameter  ParameterName=proc_control.physics.thrusters  ParameterType=double[]  ParameterMaxArrayLength=400  ParameterInitialValue=int8(zeros(1,48))  SampleTime=-1  ModelName=proc_control  BlockId=ParamGet_proc_control_194
  Volume : ros2lib/Get Parameter  ParameterName=proc_control.physics.volume  ParameterType=double  ParameterMaxArrayLength=16  ParameterInitialValue=physics.volume  SampleTime=-1  ModelName=proc_control  BlockId=ParamGet_proc_control_169
  physicsConstants : Outport
  wires:
  MATLAB System6/1 -> Bus Creator/13  "hydro_pose"
  CDL/2 -> MATLAB System1/2
  MATLAB System2/1 -> Bus Creator/9  "cdq"
  Thrusters/1 -> MATLAB Function/1(vec)
  RG/2 -> MATLAB System11/2
  CDQ/2 -> MATLAB System2/2
  Depth Pose/1 -> MATLAB System5/1
  MATLAB System8/1 -> Bus Creator/15  "dvl_rotation"
  CDL/1 -> MATLAB System1/1
  CDQ/1 -> MATLAB System2/1
  Added Mass/1 -> MATLAB System3/1
  Added Mass/2 -> MATLAB System3/2
  I/1 -> MATLAB System4/1
  I/2 -> MATLAB System4/2
  Depth Pose/2 -> MATLAB System5/2
  Hydro Pose/1 -> MATLAB System6/1
  Hydro Pose/2 -> MATLAB System6/2
  Sonar Pose/1 -> MATLAB System7/1
  Sonar Pose/2 -> MATLAB System7/2
  DVL Rotation/1 -> MATLAB System8/1
  DVL Rotation/2 -> MATLAB System8/2
  Thrusters/2 -> MATLAB Function/2(length)
  DVL Lost Override/1 -> Data Type Conversion/1
  RHO/1 -> Bus Creator/1  "rho"
  Sub Height/1 -> Bus Creator/5  "sub_height"
  G/1 -> Bus Creator/2  "g"
  Volume/1 -> Bus Creator/4  "volume"
  MATLAB System12/1 -> Bus Creator/7  "rb"
  MATLAB System1/1 -> Bus Creator/8  "cdl"
  MATLAB System3/1 -> Bus Creator/10  "added_mass"
  MATLAB System4/1 -> Bus Creator/11  "I"
  MATLAB System5/1 -> Bus Creator/12  "depth_pose"
  MATLAB System7/1 -> Bus Creator/14  "sonar_pose"
  MATLAB Function/1(array) -> Bus Creator/16  "thrusters"
  Data Type Conversion/1 -> Bus Creator/17  "dvl_lost_override"
  Bus Creator/1 -> physicsConstants/1
  Get Parameter2/1 -> Bus Creator/3  "mass"
  RG/1 -> MATLAB System11/1
  MATLAB System11/1 -> Bus Creator/6  "rg"
  RB/1 -> MATLAB System12/1
  RB/2 -> MATLAB System12/2
